simulink model "pendule_inv_etu"  (R2019a)
settings: Solver=VariableStepAuto  StartTime=0.0  StopTime=10.0  RelTol=1e-3
values from neighbouring files (symbols this model uses):
  g = 9.81    [simu_pendule_inv_capteur_etu.m]    (also in simu_pendule_inv_echant_etu.m; simu_pendule_inv_etu.m)
  l = 10    [simu_pendule_inv_capteur_etu.m]    (also in simu_pendule_inv_echant_etu.m; simu_pendule_inv_etu.m)
  ue = 0    [simu_pendule_inv_capteur_etu.m]    (also in simu_pendule_inv_echant_etu.m; simu_pendule_inv_etu.m)
  x0 = [pi/20 0]    [simu_pendule_inv_capteur_etu.m]    (also in simu_pendule_inv_echant_etu.m; simu_pendule_inv_etu.m = [pi/20 0]')
settings Model: Creator=tsadurni  LastModifiedBy=tsadurni

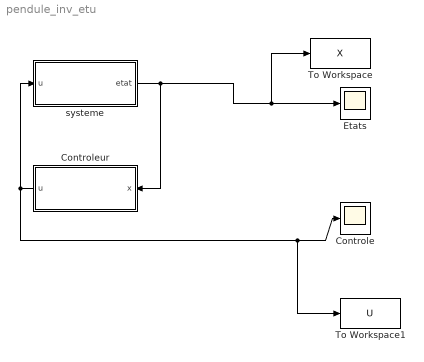
== system pendule_inv_etu ==
  "Controle " : Scope
  Controleur : Subsystem
  "Etats " : Scope
  To Workspace : ToWorkspace  VariableName=X  SaveFormat=Timeseries  SampleTime=-1
  "To Workspace1 " : ToWorkspace  VariableName=U  SaveFormat=Timeseries  SampleTime=-1
  systeme : Subsystem
  wires:
  systeme/1(etat) -> Controleur/1(x), To Workspace/1, "Etats "/1
  Controleur/1("u ") -> "To Workspace1 "/1, "Controle "/1, systeme/1(u)

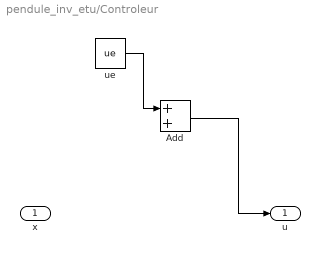
== system pendule_inv_etu/Controleur ==
  x : Inport
  Add : Sum
  "ue " : Constant  Value=ue
  "u " : Outport
  wires:
  "ue "/1 -> Add/1
  Add/1 -> "u "/1

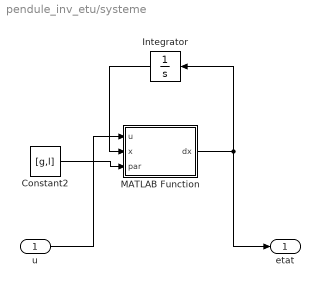
== system pendule_inv_etu/systeme ==
  u : Inport
  Constant2 : Constant  Value=[g,l]
  Integrator : Integrator  InitialCondition=x0
  MATLAB Function : MATLAB Function  TreatAsAtomicUnit=on
  etat : Outport
  wires:
  Constant2/1 -> MATLAB Function/3(par)
  u/1 -> MATLAB Function/1(u)
  MATLAB Function/1(dx) -> etat/1, Integrator/1
  Integrator/1 -> MATLAB Function/2(x)

== matlab function pendule_inv_etu/systeme/MATLAB Function ==
  data: u input; x input; dx output; par input
function dx = fcn(u,x,par)

dx = [u;x]
